simulink model "Airplane_NLSimulator"  (R2019b)
settings: Solver=ode4  StartTime=Aircraft_Data.t_i  StopTime=Aircraft_Data.t_f  FixedStep=Aircraft_Data.dt  RelTol=1e-3
PostLoadFcn:
  | %% Adding File Path to MATLAb's Search Path
  | addpath(fileparts(which(bdroot)))
  | 
  | %% Aircraft Data
  | Data_From_Excel = readmatrix('B-747 Flight Condition 5.xlsx','Range','B2:B61');
  | Aircraft_Data = AircraftData(Data_From_Excel);
  | 
  | %% Control Actions
  | Aircraft_Data.CA = [Data_From_Excel(57)*pi/180; Data_From_Excel(58)*pi/180; Data_From_Excel(59)*pi/180; Data_From_Excel(60)];
  | 
  | %% Airframe Model
  | SCDer = Airframe_Model(Aircraft_Data);
InitFcn:
  | %% Adding File Path to MATLAb's Search Path
  | addpath(fileparts(which(bdroot)))
  | 
  | %% Aircraft Data
  | Data_From_Excel = readmatrix('B-747 Flight Condition 5.xlsx','Range','B2:B61');
  | Aircraft_Data = AircraftData(Data_From_Excel);
  | 
  | %% Control Actions
  | Aircraft_Data.CA = [Data_From_Excel(57)*pi/180; Data_From_Excel(58)*pi/180; Data_From_Excel(59)*pi/180; Data_From_Excel(60)];
  | 
  | %% Airframe Model
  | SCDer = Airframe_Model(Aircraft_Data);
libraries: dspsigops x3, shared6dof x1, aerolibasang x1, sharedtransform x1
settings Model: Creator=Mahmoud A. Moustafa  LastModifiedBy=Mahmoud A. Moustafa

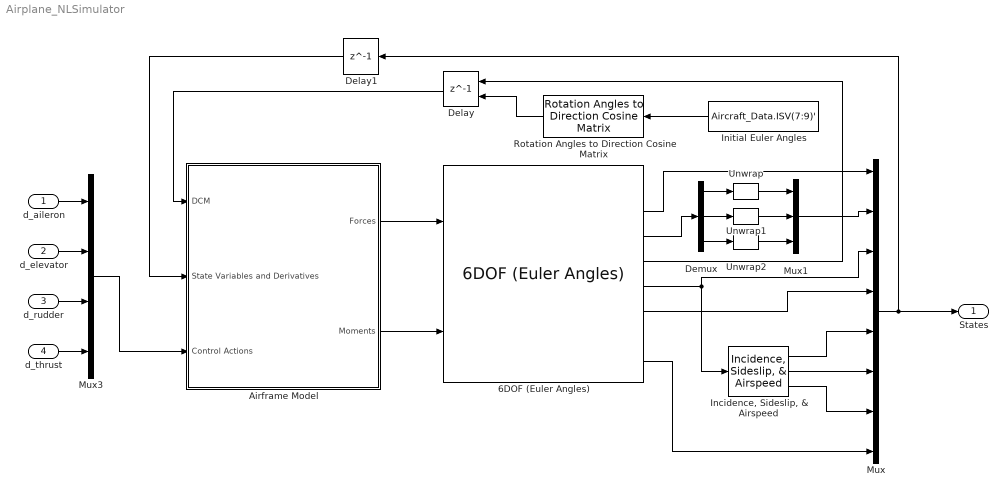
== system Airplane_NLSimulator ==
  d_aileron : Inport
  d_elevator : Inport  Port=2
  d_rudder : Inport  Port=3
  d_thrust : Inport  Port=4
  6DOF (Euler Angles) : shared6dof/6DOF (Euler Angles)  units=English (Velocity in ft/s)  mtype=Fixed  rep=Euler Angles  xme_0=Aircraft_Data.ISV(10:12)'  Vm_0=Aircraft_Data.ISV(1:3)'  eul_0=Aircraft_Data.ISV(7:9)'  pm_0=Aircraft_Data.ISV(4:6)'  mass_0=Aircraft_Data.m  mass_e=0.5  mass_f=2.0  inertia=Aircraft_Data.I  inertia_e=eye(3)  inertia_f=2*eye(3)  k_quat=1.0  vre_flag=on  abi_flag=off  aMode=0  xme_statename=''  Vm_statename=''  eul_statename=''  quat_statename=''  pm_statename=''  mass_statename=''
      settings: SourceProductBaseCode=AE
  Airframe Model : Subsystem
  Delay : Delay  DelayLength=1  InitialConditionSource=Input port  InitialCondition=0
      settings: InputPortMap=u0,p4
  Delay1 : Delay  DelayLength=1  InitialCondition=[Aircraft_Data.ISV(10:12); Aircraft_Data.ISV(7:9); Aircraft_Data.ISV(1:3); Aircraft_Data.ISV(4:6); Aircraft_Data.ISV(13:14); Aircraft_Data.V_T0; Aircraft_Data.ISD(1:3)]'
  Demux : Demux  Outputs=3
  "Incidence, Sideslip, & Airspeed" : aerolibasang/Incidence, Sideslip, & Airspeed
      settings: SourceProductName=Aerospace Blockset
  Initial Euler Angles : Constant  Value=Aircraft_Data.ISV(7:9)'
  Mux : Mux  Inputs=8
  Mux1 : Mux  Inputs=3
  Mux3 : Mux
  Rotation Angles to Direction Cosine Matrix : sharedtransform/Rotation Angles to Direction Cosine Matrix  rotationOrder=ZYX  aMode=aMode
      settings: SourceProductBaseCode=AE
  Unwrap : dspsigops/Unwrap  tol=pi  InputProcessing=Columns as channels (frame based)  running=off
  Unwrap1 : dspsigops/Unwrap  tol=pi/2  InputProcessing=Columns as channels (frame based)  running=off
  Unwrap2 : dspsigops/Unwrap  tol=pi  InputProcessing=Columns as channels (frame based)  running=off
  States : Outport
  wires:
  6DOF (Euler Angles)/5 -> Mux/3, "Incidence, Sideslip, & Airspeed"/1
  6DOF (Euler Angles)/8 -> Mux/8
  6DOF (Euler Angles)/6 -> Mux/4
  6DOF (Euler Angles)/2 -> Mux/1
  d_thrust/1 -> Mux3/4
  d_aileron/1 -> Mux3/1
  d_elevator/1 -> Mux3/2
  d_rudder/1 -> Mux3/3
  6DOF (Euler Angles)/4 -> Delay/1
  Mux/1 -> Delay1/1, States/1
  Airframe Model/1(Forces) -> 6DOF (Euler Angles)/1
  Airframe Model/2(Moments) -> 6DOF (Euler Angles)/2
  Mux3/1 -> Airframe Model/3(Control Actions)
  Delay1/1 -> Airframe Model/2(State Variables and Derivatives)
  Initial Euler Angles/1 -> Rotation Angles to Direction Cosine Matrix/1
  Delay/1 -> Airframe Model/1(DCM)
  Rotation Angles to Direction Cosine Matrix/1 -> Delay/2
  "Incidence, Sideslip, & Airspeed"/2 -> Mux/6
  "Incidence, Sideslip, & Airspeed"/1 -> Mux/5
  "Incidence, Sideslip, & Airspeed"/3 -> Mux/7
  6DOF (Euler Angles)/3 -> Demux/1
  Demux/1 -> Unwrap/1
  Demux/2 -> Unwrap1/1
  Demux/3 -> Unwrap2/1
  Unwrap/1 -> Mux1/1
  Unwrap1/1 -> Mux1/2
  Unwrap2/1 -> Mux1/3
  Mux1/1 -> Mux/2

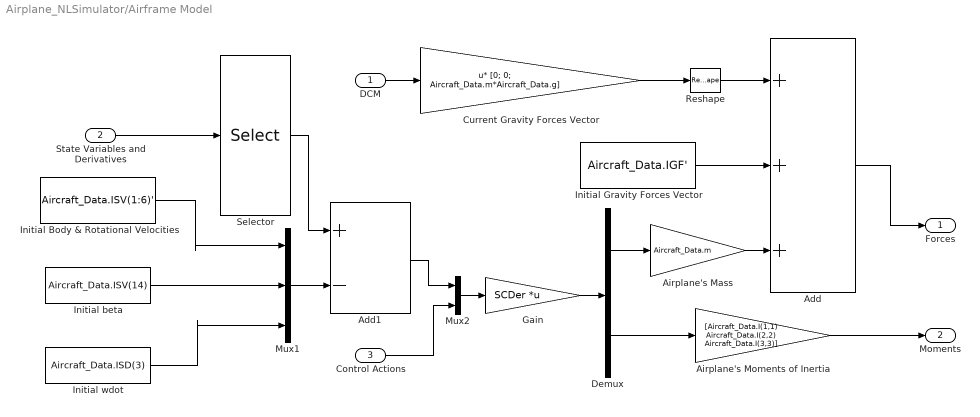
== system Airplane_NLSimulator/Airframe Model ==
  DCM : Inport
  State Variables and Derivatives : Inport  Port=2
  Control Actions : Inport  Port=3
  Add : Sum  Inputs=+++
  Add1 : Sum  Inputs=+-
  Airplane's Mass : Gain  Gain=Aircraft_Data.m
  Airplane's Moments of Inertia : Gain  Gain=[Aircraft_Data.I(1,1) Aircraft_Data.I(2,2) Aircraft_Data.I(3,3)]
  Current Gravity Forces Vector : Gain  Gain=[0; 0; Aircraft_Data.m*Aircraft_Data.g]  Multiplication=Matrix(u*K)
  Demux : Demux  Outputs=2
  Gain : Gain  Gain=SCDer  Multiplication=Matrix(K*u) (u vector)
  Initial Body & Rotational Velocities : Constant  Value=Aircraft_Data.ISV(1:6)'
  Initial Gravity Forces Vector : Constant  Value=Aircraft_Data.IGF'
  Initial beta : Constant  Value=Aircraft_Data.ISV(14)
  Initial wdot : Constant  Value=Aircraft_Data.ISD(3)
  Mux1 : Mux  Inputs=3
  Mux2 : Mux  Inputs=2
  Reshape : Reshape
  Selector : Selector  InputPortWidth=18  IndexOptions=Index vector (dialog)  Indices=[7:12 14 18]  OutputSizes=1
  Forces : Outport
  Moments : Outport  Port=2
  wires:
  Add/1 -> Forces/1
  Mux2/1 -> Gain/1
  Initial Gravity Forces Vector/1 -> Add/2
  Current Gravity Forces Vector/1 -> Reshape/1
  Selector/1 -> Add1/1
  Initial wdot/1 -> Mux1/3
  Gain/1 -> Demux/1
  Initial beta/1 -> Mux1/2
  Demux/1 -> Airplane's Mass/1
  Airplane's Mass/1 -> Add/3
  Initial Body & Rotational Velocities/1 -> Mux1/1
  Add1/1 -> Mux2/1
  Reshape/1 -> Add/1
  Demux/2 -> Airplane's Moments of Inertia/1
  Mux1/1 -> Add1/2
  Control Actions/1 -> Mux2/2
  DCM/1 -> Current Gravity Forces Vector/1
  State Variables and Derivatives/1 -> Selector/1
  Airplane's Moments of Inertia/1 -> Moments/1
